simulink model "scale_model_v3"  (R2024b)
settings: Solver=VariableStepAuto  StartTime=0.0  StopTime=100  MaxStep=0.02  RelTol=1e-3
values from neighbouring files (symbols this model uses):
  A_adrc = [zeros(N_adrc, 1)  eye(N_adrc, N_adrc) ... (first row only)    [init_scale_blade_suspendedv3.m]
  b0_adrc_roll = 15    [init_scale_blade_suspendedv3.m]
  b0_adrc_yaw = 9    [init_scale_blade_suspendedv3.m]
  b_adrc_roll = [zeros(N_adrc-1, 1) ... (first row only)    [init_scale_blade_suspendedv3.m]
  b_adrc_yaw = [zeros(N_adrc-1, 1) ... (first row only)    [init_scale_blade_suspendedv3.m]
  c_t_adrc = [1, zeros(1, N_adrc)]    [init_scale_blade_suspendedv3.m]
  eta_s_init_n = [p_s_init_n;Theta_s_init_n]    [init_scale_blade_suspended.m]    (also in init_scale_blade_suspendedv2.m; init_scale_blade_suspendedv3.m)
  g = 9.81    [init_scale_blade_suspended.m]    (also in init_scale_blade_suspendedv2.m; init_scale_blade_suspendedv3.m)
  I_s = eye(3) .*[0.0159; 0.00041299325; 0.0146]    [init_scale_blade_suspended.m]    (also in init_scale_blade_suspendedv2.m; init_scale_blade_suspendedv3.m)
  inv_M_s = inv(M_s)    [init_scale_blade_suspended.m]    (also in init_scale_blade_suspendedv2.m; init_scale_blade_suspendedv3.m)
  k_adrc = ones(N_adrc,1)    [init_scale_blade_suspendedv3.m]
  k_w1_s = gamma * EA/lw1_s_init    (= 19634.9540849)    [init_scale_blade_suspended.m]    (also in init_scale_blade_suspendedv2.m = 196349.540849; init_scale_blade_suspendedv3.m = 196349.540849)
  k_w2_s = k_w1_s    (= 19634.9540849)    [init_scale_blade_suspended.m]    (also in init_scale_blade_suspendedv2.m = 196349.540849; init_scale_blade_suspendedv3.m = 196349.540849)
  L = 0.8    [init_scale_blade_suspended.m]    (also in init_scale_blade_suspendedv2.m; init_scale_blade_suspendedv3.m)
  l_adrc = ones(N_adrc+1, 1)    [init_scale_blade_suspendedv3.m]
  lw1_s_init = tot_liftWire-0.14    (= 0.56)    [init_scale_blade_suspended.m]    (also in init_scale_blade_suspendedv2.m; init_scale_blade_suspendedv3.m)
  lw2_s = norm(p_h_s_init- posSling_s_n(:,1))-elong_lw2_s    [init_scale_blade_suspended.m]    (also in init_scale_blade_suspendedv2.m; init_scale_blade_suspendedv3.m)
  m_h_s = 0.01    [init_scale_blade_suspended.m]    (also in init_scale_blade_suspendedv2.m; init_scale_blade_suspendedv3.m)
  meanWSP = 2    [init_scale_blade_suspended.m]    (also in init_scale_blade_suspendedv2.m = 1.6; init_scale_blade_suspendedv3.m)
  N_adrc = 2    [init_scale_blade_suspendedv3.m]
  nu_s_init_b = zeros(6,1)    [init_scale_blade_suspended.m]    (also in init_scale_blade_suspendedv2.m; init_scale_blade_suspendedv3.m)
  p_h_dot_s_init = [0;0;0]    [init_scale_blade_suspended.m]    (also in init_scale_blade_suspendedv2.m; init_scale_blade_suspendedv3.m)
  p_h_s_init = posCraneTip_s + [0;0;lw1_s_init + elong_mainlw_s]    [init_scale_blade_suspended.m]    (also in init_scale_blade_suspendedv2.m; init_scale_blade_suspendedv3.m)
  posCOG_s = [0;0;0]    [init_scale_blade_suspended.m]    (also in init_scale_blade_suspendedv2.m; init_scale_blade_suspendedv3.m)
  posCraneTip_s = [0;0;-1.2]    [init_scale_blade_suspended.m]    (also in init_scale_blade_suspendedv2.m; init_scale_blade_suspendedv3.m)
  posSling_s_b = [posCOG_s + [slings_p1_new(1); -0.05; slings_p1_new(2)],                posCOG_s + [slings_p1_new(1); 0.05; slings_p1_new(2)],               posCOG_s + [slings_p2_new(1); -0.05; slings_p2_new(2)],               posCOG_s + [slings_p2_new(1); 0.05; slings_p2_new(2)]]    [init_scale_blade_suspended.m]    (also in init_scale_blade_suspendedv2.m; init_scale_blade_suspendedv3.m)
  posThruster_s_b = [posCOG_s + [0.03; 0.21; -0.05],                posCOG_s + [0.03; -0.21; -0.05],               posCOG_s + [0; 0.1825; -0.05],               posCOG_s + [0; -0.1825; -0.05]]    [init_scale_blade_suspended.m]    (also in init_scale_blade_suspendedv2.m; init_scale_blade_suspendedv3.m)
  totalMass_s = 0.391    [init_scale_blade_suspended.m]    (also in init_scale_blade_suspendedv2.m; init_scale_blade_suspendedv3.m)
  W = 0.05    [init_scale_blade_suspended.m]    (also in init_scale_blade_suspendedv2.m; init_scale_blade_suspendedv3.m)
undefined symbols (not defined in the file or in its folder): linsys_v2, sigbuilder_block
libraries: MarIn_blade x27, simulink_extras x6, simulink x1
settings Model: Creator=Basti  LastModifiedBy=Henrik
settings DebuggingCC: UnconnectedInputMsg=warning  UnconnectedOutputMsg=warning  UnconnectedLineMsg=warning
settings ModelReferenceCC: EnableRefExpFcnMdlSchedulingChecks=on
settings RTWCC: GPUComputeCapability=3.5  DLArmComputeVersion=19.05

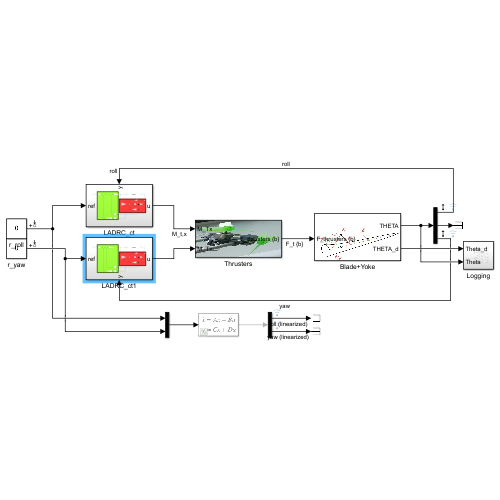
[thumbnail: Simulink's stored preview of the top-level diagram]
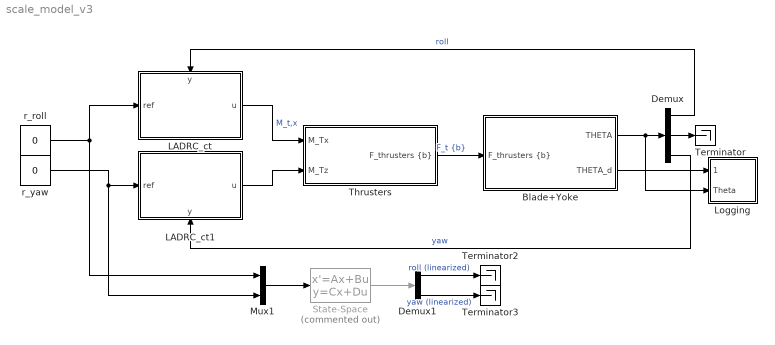
== system scale_model_v3 ==
  Blade+Yoke : Subsystem
      mask Display: image('$imagefile'); % Use "Edit Image" on toolstrip to change.
  Demux : Demux  Outputs=3
  Demux1 : Demux  Outputs=2
  LADRC_ct : Subsystem
      settings: PortSchema="{\"entries\":[{\"content\":{\"sides\":[{\"content\":{\"connectorIds\":[\"In1\"]},\"type\":\"ConnectorPlacement.EquallySpacedRectSide\",\"uuid\":\"1d520aa3-92ac-435b-91ed-fc26ef221564\"},{\"content\":{\"connectorIds\":[\"Out1\"],\"side\":\"RIGHT\"},\"type\":\"ConnectorPlacement.EquallySpacedRectSide\",\"uuid\":\"34654b5a-6fa4-4dd6-9109-9eab0d6d1617\"},{\"content\":{\"connectorIds\":[\"In2\"],\"side\":\"TOP\"},\"type\":\"ConnectorPlacement.EquallySpacedRectSide\",\"uuid\":\"33f5a30d-a2bf-471c-a0e3-d6c7b272313e\"},{\"content\":{\"side\":\"BOTTOM\"},\"type\":\"ConnectorPlacement.EquallySpacedRectSide\",\"uuid\":\"4d3b158b-a676-45c0-b7a2-124ee6e2f3af\"}]},\"type\":\"ConnectorPlacement.EquallySpacedConnector\",\"uuid\":\"f505dad7-f342-41a2-8bfc-b3754d03549d\"}],\"packageUris\":[\"http://schema.mathworks.com/mf0/Connector/R2020b\"],\"version\":\"1.0\"}"
  LADRC_ct1 : Subsystem
      settings: PortSchema="{\"entries\":[{\"content\":{\"sides\":[{\"content\":{\"connectorIds\":[\"In1\"]},\"type\":\"ConnectorPlacement.EquallySpacedRectSide\",\"uuid\":\"1d520aa3-92ac-435b-91ed-fc26ef221564\"},{\"content\":{\"connectorIds\":[\"Out1\"],\"side\":\"RIGHT\"},\"type\":\"ConnectorPlacement.EquallySpacedRectSide\",\"uuid\":\"34654b5a-6fa4-4dd6-9109-9eab0d6d1617\"},{\"content\":{\"side\":\"TOP\"},\"type\":\"ConnectorPlacement.EquallySpacedRectSide\",\"uuid\":\"33f5a30d-a2bf-471c-a0e3-d6c7b272313e\"},{\"content\":{\"connectorIds\":[\"In2\"],\"side\":\"BOTTOM\"},\"type\":\"ConnectorPlacement.EquallySpacedRectSide\",\"uuid\":\"d75252f2-61e4-4cdf-a2b4-b31b7dc5a280\"}]},\"type\":\"ConnectorPlacement.EquallySpacedConnector\",\"uuid\":\"f505dad7-f342-41a2-8bfc-b3754d03549d\"}],\"packageUris\":[\"http://schema.mathworks.com/mf0/Connector/R2020b\"],\"version\":\"1.0\"}"
  Logging : Subsystem
  Mux1 : Mux  Inputs=2
  State-Space : StateSpace  Commented=on  A=linsys_v2.A  B=linsys_v2.B  C=linsys_v2.C  D=linsys_v2.D  InitialCondition=0
  Terminator : Terminator
  Terminator2 : Terminator
  Terminator3 : Terminator
  Thrusters : Subsystem
      mask Display: image('$imagefile'); % Use "Edit Image" on toolstrip to change.
  r_roll : Constant  Value=0
  r_yaw : Constant  Value=0
  wires:
  Blade+Yoke/1(THETA) -> Demux/1, Logging/2(Theta)
  Demux/3 -> LADRC_ct1/2(y)  "yaw"
  Demux/1 -> LADRC_ct/2(y)  "roll"
  r_yaw/1 -> LADRC_ct1/1(ref), Mux1/2
  r_roll/1 -> LADRC_ct/1(ref), Mux1/1
  Thrusters/1("F_thrusters {b}") -> Blade+Yoke/1("F_thrusters {b}")  "F_t {b}"
  Blade+Yoke/2(THETA_d) -> Logging/1(Theta_d)
  Demux/2 -> Terminator/1
  Mux1/1 -> State-Space/1
  State-Space/1 -> Demux1/1
  Demux1/1 -> Terminator2/1  "roll (linearized)"
  Demux1/2 -> Terminator3/1  "yaw (linearized)"
  LADRC_ct1/1(u) -> Thrusters/2(M_Tz)
  LADRC_ct/1(u) -> Thrusters/1(M_Tx)  "M_t,x"

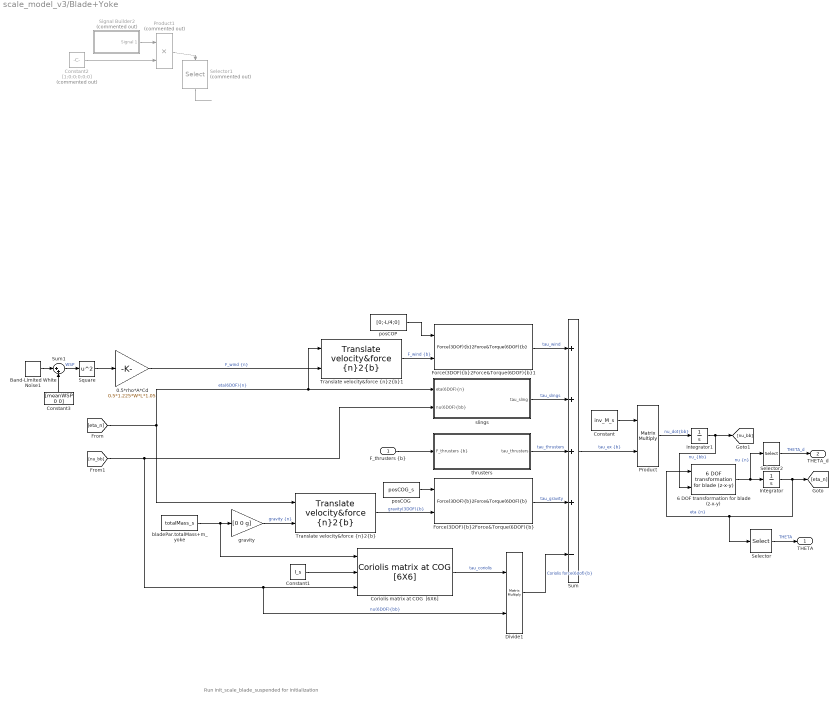
== system scale_model_v3/Blade+Yoke ==
  note: Run init_scale_blade_suspended for initialization
  "F_thrusters {b}" : Inport
  0.5*rho*A*Cd : Gain  Gain=0.5*1.225*W*L*1.05
  6 DOF transformation for blade (z-x-y) : MarIn_blade/Basic functions/6 DOF transformation for blade (z-x-y)
      settings: SourceProductName=MarIn (Blade)
  Band-Limited White Noise1 : simulink/Sources/Band-Limited White Noise  Cov=[0.001 0.001 0.001]  Ts=0.1  seed=[23321 232341 23441]
  Constant : Constant  Value=inv_M_s
  Constant1 : Constant  Value=I_s
  Constant2 : Constant  Commented=on  Value=[1;0;0;0;0;0]
  Constant3 : Constant  Value=[meanWSP 0 0]
  Coriolis matrix at COG  [6X6] : MarIn_blade/Basic functions/Coriolis matrix at COG  [6X6]
      settings: SourceProductName=MarIn (Blade)
  Divide1 : Product  Inputs=**  Multiplication=Matrix(*)
  "Force(3DOF){b}2Force&Torque(6DOF){b}" : MarIn_blade/Basic functions/Force(3DOF){b}2Force&Torque(6DOF){b}  posCOG_bb=posCOG_s
      settings: SourceProductName=MarIn (Blade)
  "Force(3DOF){b}2Force&Torque(6DOF){b}1" : MarIn_blade/Basic functions/Force(3DOF){b}2Force&Torque(6DOF){b}  posCOG_bb=posCOG_s
      settings: SourceProductName=MarIn (Blade)
  Integrator : Integrator  InitialCondition=eta_s_init_n  ContinuousStateAttributes='eta_n'
  "Integrator1 " : Integrator  InitialCondition=nu_s_init_b  ContinuousStateAttributes='nu_b'
  Product : Product  Inputs=**  Multiplication=Matrix(*)
  Product1 : Product  Commented=on
  Selector : Selector  InputPortWidth=6  IndexOptions=Index vector (dialog)  Indices=[4 5 6]  OutputSizes=1
  Selector1 : Selector  Commented=on  InputPortWidth=6  IndexOptions=Index vector (dialog)  Indices=[1 2 3]  OutputSizes=1
  Selector2 : Selector  InputPortWidth=6  IndexOptions=Index vector (dialog)  Indices=[4 5 6]  OutputSizes=1
  Signal Builder2 : Subsystem  Tag=STV Subsys  Commented=on  LoadFcn=sigbuilder_block('load');  StartFcn=sigbuilder_block('start');  StopFcn=sigbuilder_block('stop');  ClipboardFcn=sigbuilder_block('clipboard');  mask(Sigbuilder block){tuvar=[0:10]}
      mask help: Simulink:masks:SigbuilderBlock_MD
      mask init:
      | if ~strcmp(get_param(bdroot(gcbh),'SimulationStatus'),'stopped') tuvar = sigbuilder_block('maskInit'); end
      settings: CopyFcn=sigbuilder_block('copy');  DeleteFcn=sigbuilder_block('delete');  ModelCloseFcn=sigbuilder_block('modelClose');  PreSaveFcn=sigbuilder_block('preSave');  PauseFcn=sigbuilder_block('pause');  ContinueFcn=sigbuilder_block('continue');  NameChangeFcn=sigbuilder_block('namechange');  OpenFcn=sigbuilder_block('open',[437.6 199.2 550.4 400 ]);  CloseFcn=sigbuilder_block('close');
      mask Display: plot(0, 0, 100, 100,[2, 2, 32, 32, 2], [68, 8, 8, 68, 68],[32, 2], [38, 38], [32, 19, 2],[53, 60, 44], [32, 17, 17, 2],[16, 16, 31, 31]);txt = getActiveGroup(gcbh);text(2, 100, txt,'verticalAlignment', 'top');
  Square : Math  Operator=square
  Sum : Sum  Inputs=++++-
  Sum1 : Sum  Inputs=|++
  "Translate velocity&force {n}2{b}" : MarIn_blade/Basic functions/Translate velocity&force {n}2{b}
      settings: SourceProductName=MarIn (Blade)
  "Translate velocity&force {n}2{b}1" : MarIn_blade/Basic functions/Translate velocity&force {n}2{b}
      settings: SourceProductName=MarIn (Blade)
  bladePar.totalMass+m_yoke : Constant  Value=totalMass_s
  gravity : Gain  Gain=[0 0 g]
  posCOG : Constant  Value=posCOG_s
  posCOP : Constant  Value=[0;-L/4;0]
  slings : Subsystem
  thrusters : Subsystem
  THETA : Outport
  THETA_d : Outport  Port=2
  wires:
  Coriolis matrix at COG  [6X6]/1 -> Divide1/1  "tau_coriolis"
  6 DOF transformation for blade (z-x-y)/1 -> Integrator/1, Selector2/1  "nu {n}"
  "Translate velocity&force {n}2{b}"/1 -> "Force(3DOF){b}2Force&Torque(6DOF){b}"/2  "gravity(3DOF){b}"
  "Integrator1 "/1 -> [nu_bb], 6 DOF transformation for blade (z-x-y)/2  "nu_{bb}"
  "F_thrusters {b}"/1 -> thrusters/1("F_thrusters {b}")
  Sum/1 -> Product/2  "tau_ex {b}"
  Product/1 -> "Integrator1 "/1  "nu_dot{bb}"
  Integrator/1 -> [eta_n], Selector/1, 6 DOF transformation for blade (z-x-y)/1  "eta {n}"
  "Force(3DOF){b}2Force&Torque(6DOF){b}"/1 -> Sum/4  "tau_gravity"
  [eta_n] -> "Translate velocity&force {n}2{b}"/1, slings/1("eta(6DOF){n}"), "Translate velocity&force {n}2{b}1"/1  "eta(6DOF){n}"
  slings/1(tau_sling) -> Sum/2  "tau_slings"
  Constant/1 -> Product/1
  gravity/1 -> "Translate velocity&force {n}2{b}"/2  "gravity {n}"
  thrusters/1(tau_thrusters) -> Sum/3  "tau_thrusters"
  bladePar.totalMass+m_yoke/1 -> Coriolis matrix at COG  [6X6]/1, gravity/1
  [nu_bb] -> Divide1/2, Coriolis matrix at COG  [6X6]/3, slings/2("nu(6DOF){bb}")  "nu(6DOF){bb}"
  posCOG/1 -> "Force(3DOF){b}2Force&Torque(6DOF){b}"/1
  Selector/1 -> THETA/1  "THETA"
  Constant2/1 -> Product1/2
  Signal Builder2/1(Signal 1) -> Product1/1
  posCOP/1 -> "Force(3DOF){b}2Force&Torque(6DOF){b}1"/1
  "Force(3DOF){b}2Force&Torque(6DOF){b}1"/1 -> Sum/1  "tau_wind"
  0.5*rho*A*Cd/1 -> "Translate velocity&force {n}2{b}1"/2  "F_wind {n}"
  Square/1 -> 0.5*rho*A*Cd/1
  Sum1/1 -> Square/1  "WSP"
  Constant3/1 -> Sum1/2
  "Translate velocity&force {n}2{b}1"/1 -> "Force(3DOF){b}2Force&Torque(6DOF){b}1"/2  "F_wind {b}"
  Product1/1 -> Selector1/1
  Selector1/1 -> ?
  Selector2/1 -> THETA_d/1  "THETA_d"
  Band-Limited White Noise1/1 -> Sum1/1
  Constant1/1 -> Coriolis matrix at COG  [6X6]/2
  Divide1/1 -> Sum/5  "Coriolis force(6dof){b}"

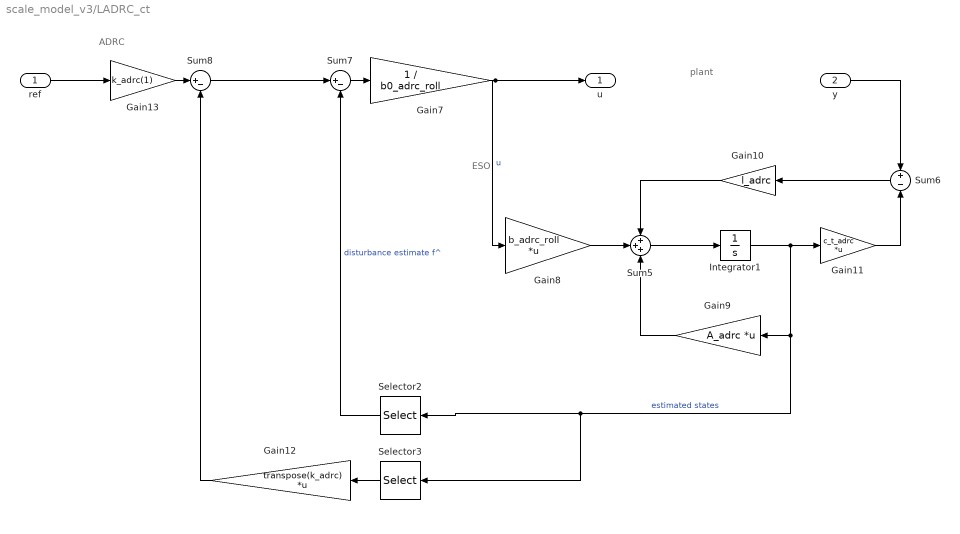
== system scale_model_v3/LADRC_ct ==
  note: plant
  note: ESO
  note: ADRC
  ref : Inport
  y : Inport  Port=2
  Gain10 : Gain  Gain=l_adrc
  Gain11 : Gain  Gain=c_t_adrc  Multiplication=Matrix(K*u)
  Gain12 : Gain  Gain=transpose(k_adrc)  Multiplication=Matrix(K*u)
  Gain13 : Gain  Gain=k_adrc(1)
  Gain7 : Gain  Gain=1 / b0_adrc_roll
  Gain8 : Gain  Gain=b_adrc_roll  Multiplication=Matrix(K*u)
  Gain9 : Gain  Gain=A_adrc  Multiplication=Matrix(K*u)
  Integrator1 : Integrator
  Selector2 : Selector  InputPortWidth=N_adrc+1  IndexOptions=Index vector (dialog)  Indices=[N_adrc+1]  OutputSizes=1
  Selector3 : Selector  InputPortWidth=N_adrc+1  IndexOptions=Index vector (dialog)  Indices=[1:N_adrc]  OutputSizes=1
  Sum5 : Sum  Inputs=+++
  Sum6 : Sum  Inputs=+|-
  Sum7 : Sum  Inputs=|+-
  Sum8 : Sum  Inputs=|+-
  u : Outport
  wires:
  Gain8/1 -> Sum5/2
  Gain7/1 -> u/1, Gain8/1  "u"
  Integrator1/1 -> Gain11/1, Selector3/1, Selector2/1, Gain9/1  "estimated states"
  Gain11/1 -> Sum6/2
  Sum6/1 -> Gain10/1
  Selector2/1 -> Sum7/2  "disturbance estimate f^"
  Sum7/1 -> Gain7/1
  Gain12/1 -> Sum8/2
  Gain10/1 -> Sum5/1
  Gain9/1 -> Sum5/3
  Gain13/1 -> Sum8/1
  Sum5/1 -> Integrator1/1
  Selector3/1 -> Gain12/1
  Sum8/1 -> Sum7/1
  ref/1 -> Gain13/1
  y/1 -> Sum6/1

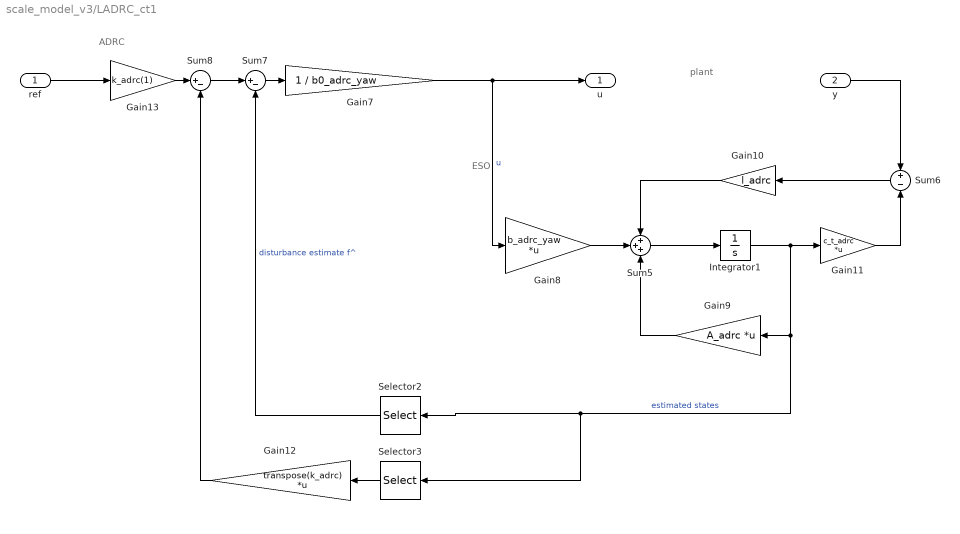
== system scale_model_v3/LADRC_ct1 ==
  note: plant
  note: ESO
  note: ADRC
  ref : Inport
  y : Inport  Port=2
  Gain10 : Gain  Gain=l_adrc
  Gain11 : Gain  Gain=c_t_adrc  Multiplication=Matrix(K*u)
  Gain12 : Gain  Gain=transpose(k_adrc)  Multiplication=Matrix(K*u)
  Gain13 : Gain  Gain=k_adrc(1)
  Gain7 : Gain  Gain=1 / b0_adrc_yaw
  Gain8 : Gain  Gain=b_adrc_yaw  Multiplication=Matrix(K*u)
  Gain9 : Gain  Gain=A_adrc  Multiplication=Matrix(K*u)
  Integrator1 : Integrator
  Selector2 : Selector  InputPortWidth=N_adrc+1  IndexOptions=Index vector (dialog)  Indices=[N_adrc+1]  OutputSizes=1
  Selector3 : Selector  InputPortWidth=N_adrc+1  IndexOptions=Index vector (dialog)  Indices=[1:N_adrc]  OutputSizes=1
  Sum5 : Sum  Inputs=+++
  Sum6 : Sum  Inputs=+|-
  Sum7 : Sum  Inputs=|+-
  Sum8 : Sum  Inputs=|+-
  u : Outport
  wires:
  Gain8/1 -> Sum5/2
  Gain7/1 -> u/1, Gain8/1  "u"
  Integrator1/1 -> Gain11/1, Selector3/1, Selector2/1, Gain9/1  "estimated states"
  Gain11/1 -> Sum6/2
  Sum6/1 -> Gain10/1
  Selector2/1 -> Sum7/2  "disturbance estimate f^"
  Sum7/1 -> Gain7/1
  Gain12/1 -> Sum8/2
  Gain10/1 -> Sum5/1
  Gain9/1 -> Sum5/3
  Gain13/1 -> Sum8/1
  Sum5/1 -> Integrator1/1
  Selector3/1 -> Gain12/1
  Sum8/1 -> Sum7/1
  ref/1 -> Gain13/1
  y/1 -> Sum6/1

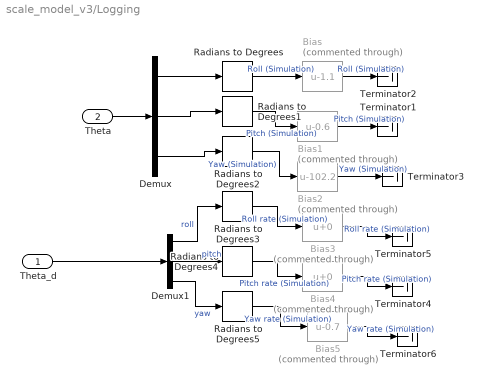
== system scale_model_v3/Logging ==
  Theta_d : Inport
  Theta : Inport  Port=2
  Bias : Bias  Commented=through  Bias=-1.1  SaturateOnIntegerOverflow=off
  Bias1 : Bias  Commented=through  Bias=-0.6  SaturateOnIntegerOverflow=off
  Bias2 : Bias  Commented=through  Bias=-102.2  SaturateOnIntegerOverflow=off
  Bias3 : Bias  Commented=through  SaturateOnIntegerOverflow=off
  Bias4 : Bias  Commented=through  SaturateOnIntegerOverflow=off
  Bias5 : Bias  Commented=through  Bias=-0.7  SaturateOnIntegerOverflow=off
  Demux : Demux  Outputs=3
  Demux1 : Demux  Outputs=3
  Radians to Degrees{,1..5} (6 alike) : simulink_extras/Transformations/Radians to Degrees
  Terminator{1..6} (6 alike) : Terminator
  wires:
  Bias5/1 -> Terminator6/1  "Yaw rate (Simulation)"
  Bias2/1 -> Terminator3/1  "Yaw (Simulation)"
  Radians to Degrees3/1 -> Bias3/1  "Roll rate (Simulation)"
  Radians to Degrees5/1 -> Bias5/1  "Yaw rate (Simulation)"
  Bias/1 -> Terminator2/1  "Roll (Simulation)"
  Radians to Degrees/1 -> Bias/1  "Roll (Simulation)"
  Bias3/1 -> Terminator5/1  "Roll rate (Simulation)"
  Radians to Degrees4/1 -> Bias4/1  "Pitch rate (Simulation)"
  Demux1/3 -> Radians to Degrees5/1  "yaw"
  Demux1/1 -> Radians to Degrees3/1  "roll"
  Radians to Degrees2/1 -> Bias2/1  "Yaw (Simulation)"
  Bias4/1 -> Terminator4/1  "Pitch rate (Simulation)"
  Bias1/1 -> Terminator1/1  "Pitch (Simulation)"
  Radians to Degrees1/1 -> Bias1/1  "Pitch (Simulation)"
  Demux1/2 -> Radians to Degrees4/1  "pitch"
  Theta_d/1 -> Demux1/1
  Theta/1 -> Demux/1
  Demux/1 -> Radians to Degrees/1
  Demux/2 -> Radians to Degrees1/1
  Demux/3 -> Radians to Degrees2/1

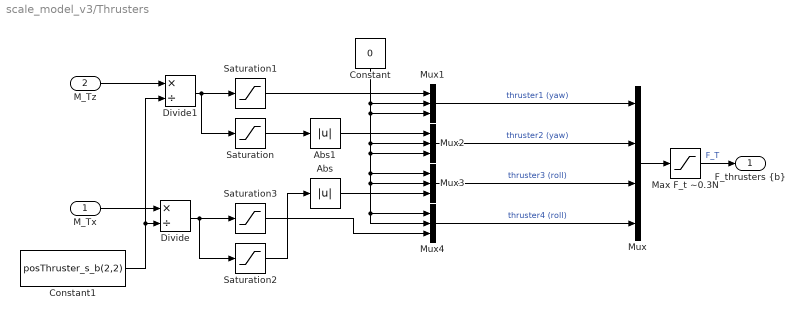
== system scale_model_v3/Thrusters ==
  M_Tx : Inport
  M_Tz : Inport  Port=2
  Abs : Abs  SaturateOnIntegerOverflow=off
  Abs1 : Abs  SaturateOnIntegerOverflow=off
  Constant : Constant  Value=0
  Constant1 : Constant  Value=posThruster_s_b(2,2)
  Divide : Product  Inputs=*/
  Divide1 : Product  Inputs=*/
  Max F_t ~0.3N : Saturate  UpperLimit=0.076  LowerLimit=-0.076  LinearizeAsGain=off
  Mux : Mux
  Mux{1..4} (4 alike) : Mux  Inputs=3
  Saturation : Saturate  UpperLimit=0  LowerLimit=-inf
  Saturation1 : Saturate  UpperLimit=inf  LowerLimit=0
  Saturation2 : Saturate  UpperLimit=0  LowerLimit=-inf
  Saturation3 : Saturate  UpperLimit=inf  LowerLimit=0
  "F_thrusters {b}" : Outport
  wires:
  Mux1/1 -> Mux/1  "thruster1 (yaw)"
  Mux2/1 -> Mux/2  "thruster2 (yaw)"
  Mux3/1 -> Mux/3  "thruster3 (roll)"
  Mux4/1 -> Mux/4  "thruster4 (roll)"
  Constant/1 -> Mux1/3, Mux3/1, Mux4/2, Mux4/1, Mux3/2, Mux2/3, Mux2/2, Mux1/2
  M_Tx/1 -> Divide/1
  Constant1/1 -> Divide1/2, Divide/2
  M_Tz/1 -> Divide1/1
  Divide1/1 -> Saturation/1, Saturation1/1
  Saturation1/1 -> Mux1/1
  Saturation/1 -> Abs1/1
  Divide/1 -> Saturation2/1, Saturation3/1
  Saturation3/1 -> Mux4/3
  Saturation2/1 -> Abs/1
  Abs/1 -> Mux3/3
  Abs1/1 -> Mux2/1
  Mux/1 -> Max F_t ~0.3N/1
  Max F_t ~0.3N/1 -> "F_thrusters {b}"/1  "F_T"

== system scale_model_v3/Blade+Yoke/Signal Builder2 ==
  Demux : Demux  Tag=STV Demux  Outputs=1
      settings: DisplayOption=none
  FromWs : FromWorkspace  Tag=STV FromWs  VariableName=tuvar
      SigBuilderData=|
      | common.afterFinalStr = 'Extrapolate'
      | common.sampleTime = 0
      | dataSet.timeRange = [0 10]
      | dataSet.name = 'Group 1'
      | sbobj.Groups.Name = 'Group 1'
      | sbobj.Groups.Signals.Name = 'Signal 1'
      | sbobj.Groups.Signals.XData = [0 2 2 2.1 2.1 10]
      | sbobj.Groups.Signals.YData = [0 0 1 1 0 0]
  Signal 1 : Outport  Tag=STV Outport
  wires:
  Demux/1 -> Signal 1/1
  FromWs/1 -> Demux/1

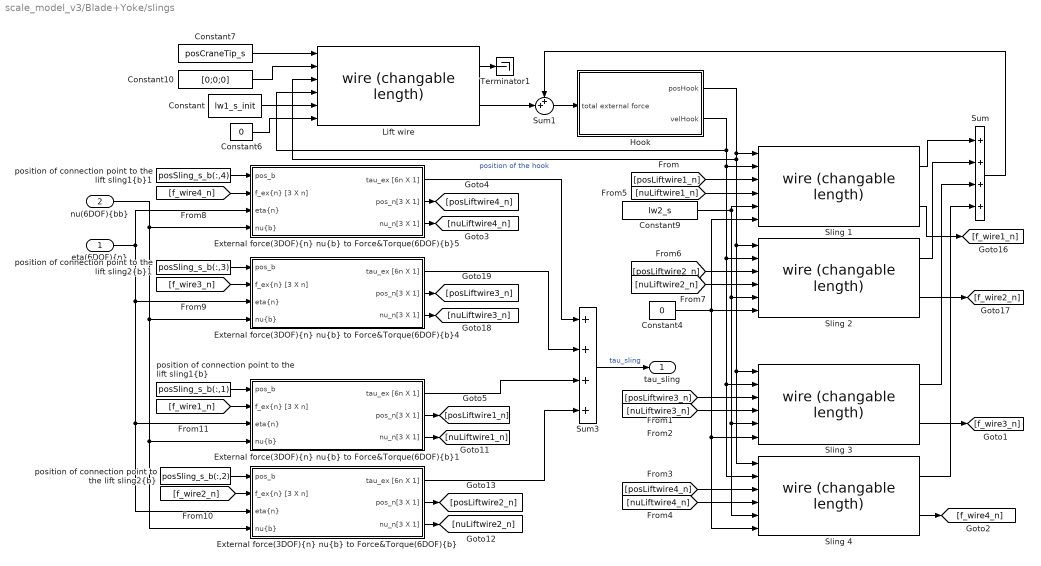
== system scale_model_v3/Blade+Yoke/slings ==
  "eta(6DOF){n}" : Inport
  "nu(6DOF){bb}" : Inport  Port=2
  Constant : Constant  Value=lw1_s_init
  Constant10 : Constant  Value=[0;0;0]
  Constant4 : Constant  Value=0
  Constant6 : Constant  Value=0
  Constant7 : Constant  Value=posCraneTip_s
  Constant9 : Constant  Value=lw2_s
  "External force(3DOF){n} nu{b} to Force&Torque(6DOF){b}" : Subsystem  AncestorBlock=MarIn_blade/Basic functions/External force(3DOF){n} nu{b} to Force&Torque(6DOF){b}  mask(External force(3DOF){n} nu{b} to Force&Torque(6DOF){b}){}
      mask help:
      | Translate position and velocity in {b} to {n}.
      |
      |
      | Author: Zhengru Ren
      | Date: April 22, 2017
  "External force(3DOF){n} nu{b} to Force&Torque(6DOF){b}1" : Subsystem  AncestorBlock=MarIn_blade/Basic functions/External force(3DOF){n} nu{b} to Force&Torque(6DOF){b}  mask(External force(3DOF){n} nu{b} to Force&Torque(6DOF){b}){}
      mask help:
      | Translate position and velocity in {b} to {n}.
      |
      |
      | Author: Zhengru Ren
      | Date: April 22, 2017
  "External force(3DOF){n} nu{b} to Force&Torque(6DOF){b}4" : Subsystem  AncestorBlock=MarIn_blade/Basic functions/External force(3DOF){n} nu{b} to Force&Torque(6DOF){b}  mask(External force(3DOF){n} nu{b} to Force&Torque(6DOF){b}){}
      mask help:
      | Translate position and velocity in {b} to {n}.
      |
      |
      | Author: Zhengru Ren
      | Date: April 22, 2017
  "External force(3DOF){n} nu{b} to Force&Torque(6DOF){b}5" : Subsystem  AncestorBlock=MarIn_blade/Basic functions/External force(3DOF){n} nu{b} to Force&Torque(6DOF){b}  mask(External force(3DOF){n} nu{b} to Force&Torque(6DOF){b}){}
      mask help:
      | Translate position and velocity in {b} to {n}.
      |
      |
      | Author: Zhengru Ren
      | Date: April 22, 2017
  Hook : Subsystem  AncestorBlock=|  mask(Hook){m_h=m_h_s, p_h_init=p_h_s_init, p_h_dot_init=p_h_dot_s_init}
      | MarIn_blade/Lifting equipments
      | (winch, wire, hook)/Hook
      mask prompts: m_h "Hook mass (m_h) [kg]"; p_h_init "Initial position of the hook"; p_h_dot_init "Initial velocity of the hook"
      mask help:
      | Used to simulate a hook.
      |
      | Author: Zhengru Ren
      | Date: May 20, 2016
      mask init:
      | invM_h = diag([1/m_h,1/m_h,1/m_h]);
  Lift wire : MarIn_blade/Lifting equipments (winch, wire, hook)/wire (changable length)  k=k_w1_s  c=d_w1_s
      settings: SourceProductName=MarIn (Blade)
  Sling {1..4} (4 alike) : MarIn_blade/Lifting equipments (winch, wire, hook)/wire (changable length)  k=k_w2_s  c=d_w2_s
      settings: SourceProductName=MarIn (Blade)
  Sum : Sum  Inputs=++++
  Sum1 : Sum  Inputs=++|
  Sum3 : Sum  Inputs=4
  Terminator1 : Terminator
  "position of connection point to the lift sling1{b}" : Constant  Value=posSling_s_b(:,1)
  "position of connection point to the lift sling1{b}1" : Constant  Value=posSling_s_b(:,4)
  "position of connection point to the lift sling2{b}" : Constant  Value=posSling_s_b(:,2)
  "position of connection point to the lift sling2{b}1" : Constant  Value=posSling_s_b(:,3)
  tau_sling : Outport
  wires:
  "nu(6DOF){bb}"/1 -> "External force(3DOF){n} nu{b} to Force&Torque(6DOF){b}"/4("nu{b}"), "External force(3DOF){n} nu{b} to Force&Torque(6DOF){b}1"/4("nu{b}"), "External force(3DOF){n} nu{b} to Force&Torque(6DOF){b}4"/4("nu{b}"), "External force(3DOF){n} nu{b} to Force&Torque(6DOF){b}5"/4("nu{b}")
  "position of connection point to the lift sling1{b}1"/1 -> "External force(3DOF){n} nu{b} to Force&Torque(6DOF){b}5"/1(pos_b)
  "External force(3DOF){n} nu{b} to Force&Torque(6DOF){b}"/1(tau_ex [6n X 1]) -> Sum3/4
  "eta(6DOF){n}"/1 -> "External force(3DOF){n} nu{b} to Force&Torque(6DOF){b}5"/3("eta{n}"), "External force(3DOF){n} nu{b} to Force&Torque(6DOF){b}"/3("eta{n}"), "External force(3DOF){n} nu{b} to Force&Torque(6DOF){b}1"/3("eta{n}"), "External force(3DOF){n} nu{b} to Force&Torque(6DOF){b}4"/3("eta{n}")
  "External force(3DOF){n} nu{b} to Force&Torque(6DOF){b}5"/1(tau_ex [6n X 1]) -> Sum3/1
  "position of connection point to the lift sling2{b}"/1 -> "External force(3DOF){n} nu{b} to Force&Torque(6DOF){b}"/1(pos_b)
  Sum3/1 -> tau_sling/1  "tau_sling"
  "External force(3DOF){n} nu{b} to Force&Torque(6DOF){b}4"/1(tau_ex [6n X 1]) -> Sum3/2
  [f_wire4_n] -> "External force(3DOF){n} nu{b} to Force&Torque(6DOF){b}5"/2("f_ex{n} [3 X n]")
  [f_wire3_n] -> "External force(3DOF){n} nu{b} to Force&Torque(6DOF){b}4"/2("f_ex{n} [3 X n]")
  "position of connection point to the lift sling2{b}1"/1 -> "External force(3DOF){n} nu{b} to Force&Torque(6DOF){b}4"/1(pos_b)
  "External force(3DOF){n} nu{b} to Force&Torque(6DOF){b}1"/3(nu_n[3 X 1]) -> [nuLiftwire1_n]
  "External force(3DOF){n} nu{b} to Force&Torque(6DOF){b}4"/2(pos_n[3 X 1]) -> [posLiftwire3_n]
  "position of connection point to the lift sling1{b}"/1 -> "External force(3DOF){n} nu{b} to Force&Torque(6DOF){b}1"/1(pos_b)
  "External force(3DOF){n} nu{b} to Force&Torque(6DOF){b}4"/3(nu_n[3 X 1]) -> [nuLiftwire3_n]
  [f_wire2_n] -> "External force(3DOF){n} nu{b} to Force&Torque(6DOF){b}"/2("f_ex{n} [3 X n]")
  "External force(3DOF){n} nu{b} to Force&Torque(6DOF){b}"/3(nu_n[3 X 1]) -> [nuLiftwire2_n]
  "External force(3DOF){n} nu{b} to Force&Torque(6DOF){b}"/2(pos_n[3 X 1]) -> [posLiftwire2_n]
  "External force(3DOF){n} nu{b} to Force&Torque(6DOF){b}1"/1(tau_ex [6n X 1]) -> Sum3/3
  "External force(3DOF){n} nu{b} to Force&Torque(6DOF){b}1"/2(pos_n[3 X 1]) -> [posLiftwire1_n]
  [f_wire1_n] -> "External force(3DOF){n} nu{b} to Force&Torque(6DOF){b}1"/2("f_ex{n} [3 X n]")
  Sling 4/2 -> [f_wire4_n]
  Sling 3/2 -> [f_wire3_n]
  Sling 4/1 -> Sum/4
  Sling 3/1 -> Sum/3
  [posLiftwire3_n] -> Sling 3/3
  [nuLiftwire3_n] -> Sling 3/4
  Hook/2(velHook) -> Sling 3/2, Sling 4/2, Sling 2/2, Sling 1/2, Lift wire/4
  Constant/1 -> Lift wire/5
  [posLiftwire1_n] -> Sling 1/3
  Sling 1/2 -> [f_wire1_n]
  [nuLiftwire1_n] -> Sling 1/4
  Sling 2/1 -> Sum/2
  Sling 2/2 -> [f_wire2_n]
  [posLiftwire2_n] -> Sling 2/3
  [nuLiftwire2_n] -> Sling 2/4
  Constant9/1 -> Sling 1/5, Sling 2/5, Sling 3/5, Sling 4/5
  Constant7/1 -> Lift wire/1
  Constant10/1 -> Lift wire/2
  Sum/1 -> Sum1/1
  Lift wire/2 -> Sum1/2
  Lift wire/1 -> Terminator1/1
  Sum1/1 -> Hook/1(total external force)
  Hook/1(posHook) -> Sling 3/1, Sling 4/1, Sling 2/1, Lift wire/3, Sling 1/1  "position of the hook"
  Constant4/1 -> Sling 2/6, Sling 1/6, Sling 3/6, Sling 4/6
  Constant6/1 -> Lift wire/6
  Sling 1/1 -> Sum/1
  [nuLiftwire4_n] -> Sling 4/4
  [posLiftwire4_n] -> Sling 4/3
  "External force(3DOF){n} nu{b} to Force&Torque(6DOF){b}5"/3(nu_n[3 X 1]) -> [nuLiftwire4_n]
  "External force(3DOF){n} nu{b} to Force&Torque(6DOF){b}5"/2(pos_n[3 X 1]) -> [posLiftwire4_n]

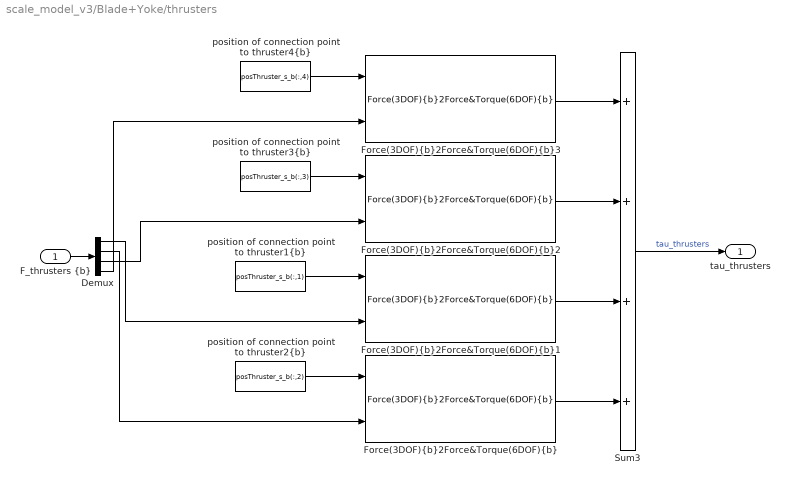
== system scale_model_v3/Blade+Yoke/thrusters ==
  "F_thrusters {b}" : Inport
  Demux : Demux
  Force(3DOF){b}2Force&Torque(6DOF){b}{,1..3} (4 alike) : MarIn_blade/Basic functions/Force(3DOF){b}2Force&Torque(6DOF){b}  posCOG_bb=posCOG_s
      settings: SourceProductName=MarIn (Blade)
  Sum3 : Sum  Inputs=4
  "position of connection point to thruster1{b}" : Constant  Value=posThruster_s_b(:,1)
  "position of connection point to thruster2{b}" : Constant  Value=posThruster_s_b(:,2)
  "position of connection point to thruster3{b}" : Constant  Value=posThruster_s_b(:,3)
  "position of connection point to thruster4{b}" : Constant  Value=posThruster_s_b(:,4)
  tau_thrusters : Outport
  wires:
  "position of connection point to thruster1{b}"/1 -> "Force(3DOF){b}2Force&Torque(6DOF){b}1"/1
  "position of connection point to thruster3{b}"/1 -> "Force(3DOF){b}2Force&Torque(6DOF){b}2"/1
  Sum3/1 -> tau_thrusters/1  "tau_thrusters"
  "position of connection point to thruster2{b}"/1 -> "Force(3DOF){b}2Force&Torque(6DOF){b}"/1
  "Force(3DOF){b}2Force&Torque(6DOF){b}"/1 -> Sum3/4
  "position of connection point to thruster4{b}"/1 -> "Force(3DOF){b}2Force&Torque(6DOF){b}3"/1
  "Force(3DOF){b}2Force&Torque(6DOF){b}3"/1 -> Sum3/1
  "Force(3DOF){b}2Force&Torque(6DOF){b}2"/1 -> Sum3/2
  "Force(3DOF){b}2Force&Torque(6DOF){b}1"/1 -> Sum3/3
  "F_thrusters {b}"/1 -> Demux/1
  Demux/4 -> "Force(3DOF){b}2Force&Torque(6DOF){b}3"/2
  Demux/3 -> "Force(3DOF){b}2Force&Torque(6DOF){b}2"/2
  Demux/1 -> "Force(3DOF){b}2Force&Torque(6DOF){b}1"/2
  Demux/2 -> "Force(3DOF){b}2Force&Torque(6DOF){b}"/2

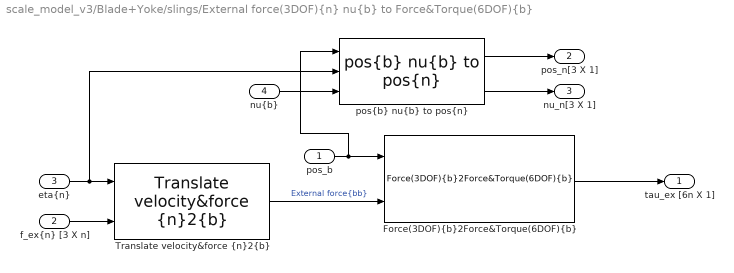
== system scale_model_v3/Blade+Yoke/slings/External force(3DOF){n} nu{b} to Force&Torque(6DOF){b} ==
  pos_b : Inport
  "f_ex{n} [3 X n]" : Inport  Port=2
  "eta{n}" : Inport  Port=3
  "nu{b}" : Inport  Port=4
  "Force(3DOF){b}2Force&Torque(6DOF){b}" : MarIn_blade/Basic functions/Force(3DOF){b}2Force&Torque(6DOF){b}  posCOG_bb=posCOG_s
      settings: SourceProductName=MarIn (Blade)
  "Translate velocity&force {n}2{b}" : MarIn_blade/Basic functions/Translate velocity&force {n}2{b}
      settings: SourceProductName=MarIn (Blade)
  "pos{b} nu{b} to pos{n}" : MarIn_blade/Basic functions/pos{b} nu{b} to pos{n}  posCOG_bb=posCOG_s
      settings: SourceProductName=MarIn (Blade)
  tau_ex [6n X 1] : Outport
  pos_n[3 X 1] : Outport  Port=2
  nu_n[3 X 1] : Outport  Port=3
  wires:
  "eta{n}"/1 -> "Translate velocity&force {n}2{b}"/1, "pos{b} nu{b} to pos{n}"/2
  "f_ex{n} [3 X n]"/1 -> "Translate velocity&force {n}2{b}"/2
  "Force(3DOF){b}2Force&Torque(6DOF){b}"/1 -> tau_ex [6n X 1]/1
  "Translate velocity&force {n}2{b}"/1 -> "Force(3DOF){b}2Force&Torque(6DOF){b}"/2  "External force{bb}"
  pos_b/1 -> "Force(3DOF){b}2Force&Torque(6DOF){b}"/1, "pos{b} nu{b} to pos{n}"/1
  "pos{b} nu{b} to pos{n}"/1 -> pos_n[3 X 1]/1
  "nu{b}"/1 -> "pos{b} nu{b} to pos{n}"/3
  "pos{b} nu{b} to pos{n}"/2 -> nu_n[3 X 1]/1

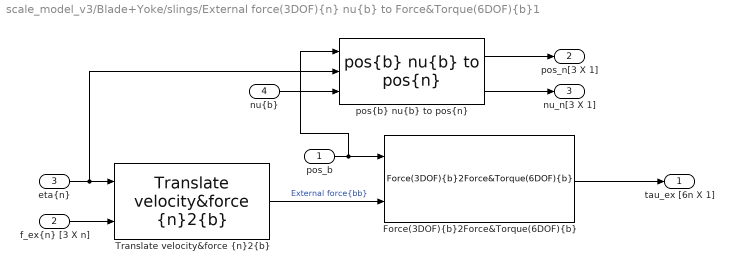
== system scale_model_v3/Blade+Yoke/slings/External force(3DOF){n} nu{b} to Force&Torque(6DOF){b}1 ==
  pos_b : Inport
  "f_ex{n} [3 X n]" : Inport  Port=2
  "eta{n}" : Inport  Port=3
  "nu{b}" : Inport  Port=4
  "Force(3DOF){b}2Force&Torque(6DOF){b}" : MarIn_blade/Basic functions/Force(3DOF){b}2Force&Torque(6DOF){b}  posCOG_bb=posCOG_s
      settings: SourceProductName=MarIn (Blade)
  "Translate velocity&force {n}2{b}" : MarIn_blade/Basic functions/Translate velocity&force {n}2{b}
      settings: SourceProductName=MarIn (Blade)
  "pos{b} nu{b} to pos{n}" : MarIn_blade/Basic functions/pos{b} nu{b} to pos{n}  posCOG_bb=posCOG_s
      settings: SourceProductName=MarIn (Blade)
  tau_ex [6n X 1] : Outport
  pos_n[3 X 1] : Outport  Port=2
  nu_n[3 X 1] : Outport  Port=3
  wires:
  "eta{n}"/1 -> "Translate velocity&force {n}2{b}"/1, "pos{b} nu{b} to pos{n}"/2
  "f_ex{n} [3 X n]"/1 -> "Translate velocity&force {n}2{b}"/2
  "Force(3DOF){b}2Force&Torque(6DOF){b}"/1 -> tau_ex [6n X 1]/1
  "Translate velocity&force {n}2{b}"/1 -> "Force(3DOF){b}2Force&Torque(6DOF){b}"/2  "External force{bb}"
  pos_b/1 -> "Force(3DOF){b}2Force&Torque(6DOF){b}"/1, "pos{b} nu{b} to pos{n}"/1
  "pos{b} nu{b} to pos{n}"/1 -> pos_n[3 X 1]/1
  "nu{b}"/1 -> "pos{b} nu{b} to pos{n}"/3
  "pos{b} nu{b} to pos{n}"/2 -> nu_n[3 X 1]/1

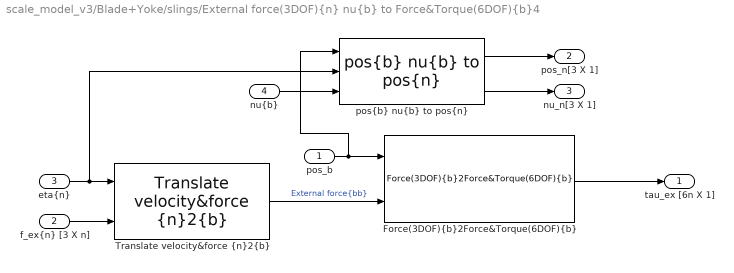
== system scale_model_v3/Blade+Yoke/slings/External force(3DOF){n} nu{b} to Force&Torque(6DOF){b}4 ==
  pos_b : Inport
  "f_ex{n} [3 X n]" : Inport  Port=2
  "eta{n}" : Inport  Port=3
  "nu{b}" : Inport  Port=4
  "Force(3DOF){b}2Force&Torque(6DOF){b}" : MarIn_blade/Basic functions/Force(3DOF){b}2Force&Torque(6DOF){b}  posCOG_bb=posCOG_s
      settings: SourceProductName=MarIn (Blade)
  "Translate velocity&force {n}2{b}" : MarIn_blade/Basic functions/Translate velocity&force {n}2{b}
      settings: SourceProductName=MarIn (Blade)
  "pos{b} nu{b} to pos{n}" : MarIn_blade/Basic functions/pos{b} nu{b} to pos{n}  posCOG_bb=posCOG_s
      settings: SourceProductName=MarIn (Blade)
  tau_ex [6n X 1] : Outport
  pos_n[3 X 1] : Outport  Port=2
  nu_n[3 X 1] : Outport  Port=3
  wires:
  "eta{n}"/1 -> "Translate velocity&force {n}2{b}"/1, "pos{b} nu{b} to pos{n}"/2
  "f_ex{n} [3 X n]"/1 -> "Translate velocity&force {n}2{b}"/2
  "Force(3DOF){b}2Force&Torque(6DOF){b}"/1 -> tau_ex [6n X 1]/1
  "Translate velocity&force {n}2{b}"/1 -> "Force(3DOF){b}2Force&Torque(6DOF){b}"/2  "External force{bb}"
  pos_b/1 -> "Force(3DOF){b}2Force&Torque(6DOF){b}"/1, "pos{b} nu{b} to pos{n}"/1
  "pos{b} nu{b} to pos{n}"/1 -> pos_n[3 X 1]/1
  "nu{b}"/1 -> "pos{b} nu{b} to pos{n}"/3
  "pos{b} nu{b} to pos{n}"/2 -> nu_n[3 X 1]/1

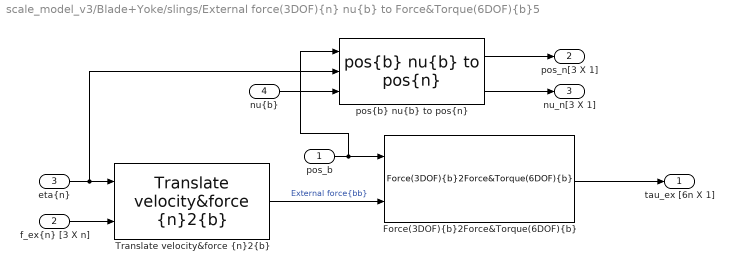
== system scale_model_v3/Blade+Yoke/slings/External force(3DOF){n} nu{b} to Force&Torque(6DOF){b}5 ==
  pos_b : Inport
  "f_ex{n} [3 X n]" : Inport  Port=2
  "eta{n}" : Inport  Port=3
  "nu{b}" : Inport  Port=4
  "Force(3DOF){b}2Force&Torque(6DOF){b}" : MarIn_blade/Basic functions/Force(3DOF){b}2Force&Torque(6DOF){b}  posCOG_bb=posCOG_s
      settings: SourceProductName=MarIn (Blade)
  "Translate velocity&force {n}2{b}" : MarIn_blade/Basic functions/Translate velocity&force {n}2{b}
      settings: SourceProductName=MarIn (Blade)
  "pos{b} nu{b} to pos{n}" : MarIn_blade/Basic functions/pos{b} nu{b} to pos{n}  posCOG_bb=posCOG_s
      settings: SourceProductName=MarIn (Blade)
  tau_ex [6n X 1] : Outport
  pos_n[3 X 1] : Outport  Port=2
  nu_n[3 X 1] : Outport  Port=3
  wires:
  "eta{n}"/1 -> "Translate velocity&force {n}2{b}"/1, "pos{b} nu{b} to pos{n}"/2
  "f_ex{n} [3 X n]"/1 -> "Translate velocity&force {n}2{b}"/2
  "Force(3DOF){b}2Force&Torque(6DOF){b}"/1 -> tau_ex [6n X 1]/1
  "Translate velocity&force {n}2{b}"/1 -> "Force(3DOF){b}2Force&Torque(6DOF){b}"/2  "External force{bb}"
  pos_b/1 -> "Force(3DOF){b}2Force&Torque(6DOF){b}"/1, "pos{b} nu{b} to pos{n}"/1
  "pos{b} nu{b} to pos{n}"/1 -> pos_n[3 X 1]/1
  "nu{b}"/1 -> "pos{b} nu{b} to pos{n}"/3
  "pos{b} nu{b} to pos{n}"/2 -> nu_n[3 X 1]/1

== system scale_model_v3/Blade+Yoke/slings/Hook ==
  total external force : Inport
  Integrator2 : Integrator  InitialCondition=p_h_dot_init  ContinuousStateAttributes='nu_hook'
  Integrator3 : Integrator  InitialCondition=p_h_init  ContinuousStateAttributes='pos_hook'
  Sum6 : Sum
  hook gravity : Constant  Value=[0;0;m_h*g]
  invM_h : Gain  Gain=invM_h  Multiplication=Matrix(K*u)
  posHook : Outport
  velHook : Outport  Port=2
  wires:
  Integrator2/1 -> velHook/1, Integrator3/1  "p_h_dot"
  total external force/1 -> Sum6/1
  hook gravity/1 -> Sum6/2
  invM_h/1 -> Integrator2/1  "p_h_ddot"
  Sum6/1 -> invM_h/1
  Integrator3/1 -> posHook/1  "p_h"
